simulink model "FM_Broadcast_Receiver"  (R2022a)
settings: Solver=FixedStepDiscrete  StartTime=0.0  StopTime=inf  RelTol=1e-3
PreLoadFcn:
  | addpath('matlab/broadcast');
undefined symbols (not defined in the file): fdesignblkfcn, gcbh
libraries: dspsigops x4, dsparch4 x4, dspsnks4 x1, sdrrlib x1
settings Model: Creator=Kate  LastModifiedBy=vovan
settings SolverCC: AlgebraicLoopSolver=TrustRegion
settings DebuggingCC: UnconnectedInputMsg=warning  UnconnectedOutputMsg=warning  UnconnectedLineMsg=warning  SFMachineParentedDataDiag=warning
settings SFSimCC: CustomCodeUndefinedFunction=UseInterfaceOnly

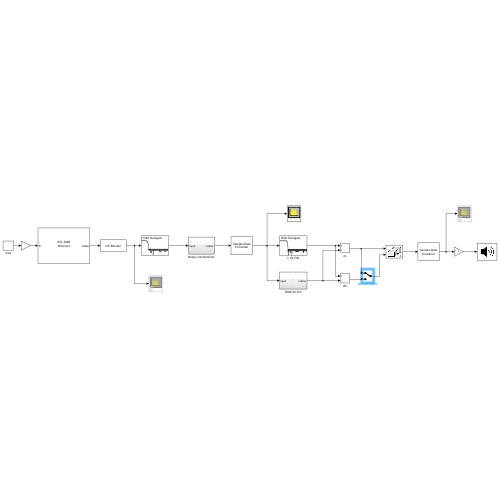
[thumbnail: Simulink's stored preview of the top-level diagram]
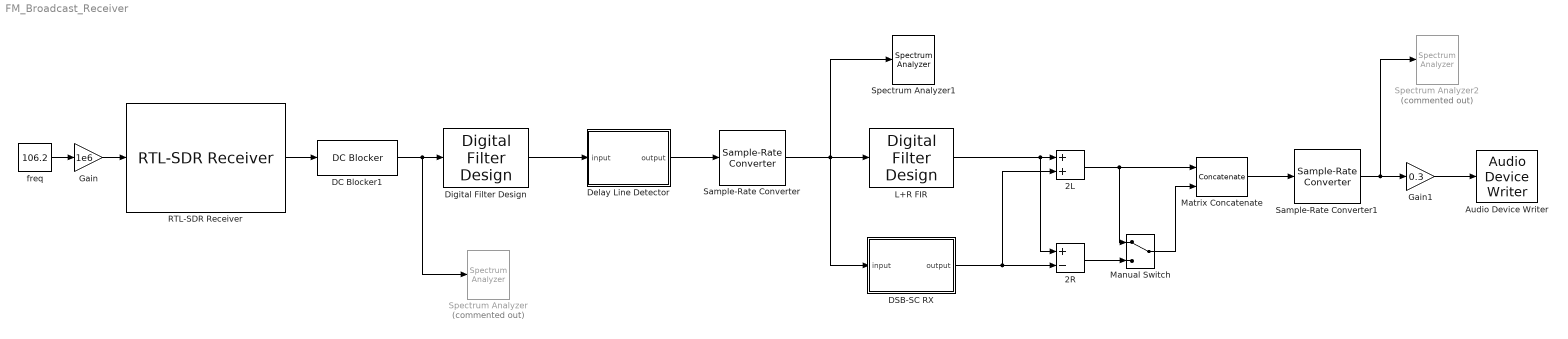
== system FM_Broadcast_Receiver ==
  2L : Sum
  2R : Sum  Inputs=+-
  Audio Device Writer : dspsnks4/Audio Device Writer  Driver=ALSA  Device=Default  InheritSampleRate=on  SampleRate=44100  BitDepth=16-bit integer  BufferSize=4096  NumBuffers=10  DefaultOutputChannelMapping=on  OutputChannelMapping=1:2  OutputNumUnderrunSamples=off  DriverIdx=8  DeviceWarnFlag=''
  DC Blocker1 : dspsigops/DC Blocker  Algorithm=IIR  NormalizedBandwidth=0.001  Length=50  Order=6  SimulateUsing=Code generation
      settings: SourceProductBaseCode=DS
  DSB-SC RX : Subsystem
  Delay Line Detector : Subsystem
  Digital Filter Design : dsparch4/Digital Filter Design  mwdsp_browser_bugfix_var=off
  Gain : Gain  Gain=1e6
  Gain1 : Gain  Gain=0.3
  L+R FIR : dsparch4/Digital Filter Design  mwdsp_browser_bugfix_var=off
  Manual Switch : ManualSwitch
  Matrix Concatenate : Concatenate  Mode=Multidimensional array  ConcatenateDimension=2
  RTL-SDR Receiver : sdrrlib/RTL-SDR Receiver  IPAddress=0  CenterFrequencySource=Input port  CenterFrequency=102.5e6  GainSource=AGC  Gain=0  ADCRate=1.2e6  FrequencyCorrection=0  LostSamplesOutputPort=off  LatencyOutputPort=off  OutputDataType=double  FrameLength=512*25  EnableBurstMode=off  NumFramesInBurst=20  sobjType=sdrr.internal.SDRRTLReceiverSL  dataUDPPort=-1  ctrlUDPPort=-1  subDeviceList=nosubdev  sdrBlockType=SDRBlockTypeSLT.SDRRxBlock  requester=UNUSED_BY_SFCN  sdrExecutionMode=SDRExecutionModeSLT.ExecModeHW  BypassUserLogic=off  DecimatorSelect=DDC decimator  SourceSelect=RF data  SineAmplitude=16000  EnableInternalClock=off  BypassIQBalance=off  IFBandwidth=40e6  ADCRateSource=Dialog  IntermediateFrequency=0  DecimationFactorSource=Dialog  DecimationFactor=512  RFFrequencyIsTunable=logical(1)  SampleTime=(512*25)/(1.2e6)  IFBandwidthSource=Dialog  SineFrequency=30000  BypassDCBlockingFilter=off  IntermediateFrequencySource=Dialog  IQBalanceCoefficients=64  SkipAllHardwareResetAndInitialization=off  EnableIQCalibrationTable=on  CacheIQCalibrationTable=off  EnableOffsetTuning=off  EnableRTLAGC=off  EnableTestMode=off  EnableTunerAGC=on  FrequencyCorrectionSource=Dialog  NumMLBuffers=128  NumUSBBuffers=16  RTLCrystalFrequency=28800000  TunerCrystalFrequency=28800000
      settings: SourceProductBaseCode=RTLSDR
  Sample-Rate Converter : dspsigops/Sample-Rate Converter  InputSampleRate=1.2e6  OutputSampleRate=1.2e5  OutputRateTolerance=0  Bandwidth=1.1e5  StopbandAttenuation=80  SimulateUsing=Code generation
      settings: SourceProductBaseCode=DS
  Sample-Rate Converter1 : dspsigops/Sample-Rate Converter  InputSampleRate=1.2e5  OutputSampleRate=48e3  OutputRateTolerance=0  Bandwidth=30e3  StopbandAttenuation=80  SimulateUsing=Code generation
      settings: SourceProductBaseCode=DS
  Spectrum Analyzer : SpectrumAnalyzer  Commented=on
  Spectrum Analyzer1 : SpectrumAnalyzer
  Spectrum Analyzer2 : SpectrumAnalyzer  Commented=on
  freq : Constant  Value=106.2
  wires:
  freq/1 -> Gain/1
  Gain/1 -> RTL-SDR Receiver/1
  Gain1/1 -> Audio Device Writer/1
  RTL-SDR Receiver/1 -> DC Blocker1/1
  DC Blocker1/1 -> Spectrum Analyzer/1, Digital Filter Design/1
  Sample-Rate Converter1/1 -> Spectrum Analyzer2/1, Gain1/1
  Digital Filter Design/1 -> Delay Line Detector/1(input)
  Delay Line Detector/1(output) -> Sample-Rate Converter/1
  Sample-Rate Converter/1 -> Spectrum Analyzer1/1, L+R FIR/1, DSB-SC RX/1(input)
  L+R FIR/1 -> 2R/1, 2L/1
  2L/1 -> Manual Switch/1, Matrix Concatenate/1
  Matrix Concatenate/1 -> Sample-Rate Converter1/1
  2R/1 -> Manual Switch/2
  Manual Switch/1 -> Matrix Concatenate/2
  DSB-SC RX/1(output) -> 2R/2, 2L/2

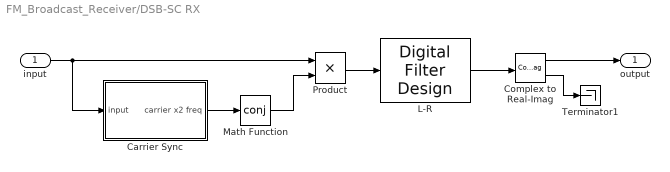
== system FM_Broadcast_Receiver/DSB-SC RX ==
  input : Inport
  Carrier Sync : Subsystem
  Complex to Real-Imag : ComplexToRealImag
  L-R : dsparch4/Digital Filter Design  mwdsp_browser_bugfix_var=off
  Math Function : Math  Operator=conj
  Product : Product
  Terminator1 : Terminator
  output : Outport
  wires:
  Carrier Sync/1(carrier x2 freq) -> Math Function/1
  Complex to Real-Imag/2 -> Terminator1/1
  L-R/1 -> Complex to Real-Imag/1
  Math Function/1 -> Product/2
  Complex to Real-Imag/1 -> output/1
  Product/1 -> L-R/1
  input/1 -> Product/1, Carrier Sync/1(input)

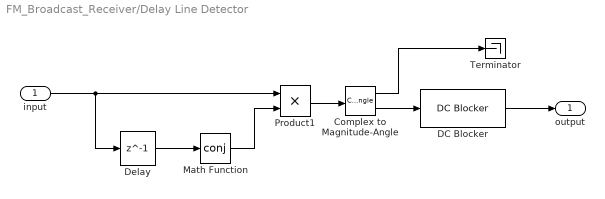
== system FM_Broadcast_Receiver/Delay Line Detector ==
  input : Inport
  Complex to Magnitude-Angle : ComplexToMagnitudeAngle
  DC Blocker : dspsigops/DC Blocker  Algorithm=IIR  NormalizedBandwidth=0.001  Length=50  Order=6  SimulateUsing=Code generation
      settings: SourceProductBaseCode=DS
  Delay : Delay  DelayLength=1  InputProcessing=Columns as channels (frame based)
  Math Function : Math  Operator=conj  SignedPower=on
  Product1 : Product
  Terminator : Terminator
  output : Outport
  wires:
  Complex to Magnitude-Angle/1 -> Terminator/1
  Math Function/1 -> Product1/2
  Complex to Magnitude-Angle/2 -> DC Blocker/1
  Delay/1 -> Math Function/1
  input/1 -> Product1/1, Delay/1
  Product1/1 -> Complex to Magnitude-Angle/1
  DC Blocker/1 -> output/1

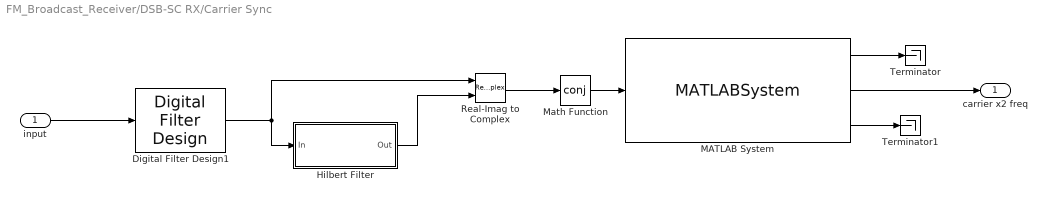
== system FM_Broadcast_Receiver/DSB-SC RX/Carrier Sync ==
  input : Inport
  Digital Filter Design1 : dsparch4/Digital Filter Design  mwdsp_browser_bugfix_var=off
  Hilbert Filter : Subsystem  DialogController=fdesignblkfcn  InitFcn=fdesignblkfcn(gcbh, {'InitFcn'});  mask(Hilbert Filter){}
      mask help: Design a Hilbert filter
      settings: CopyFcn=fdesignblkfcn(gcbh, {'CopyFcn'});
      mask Help: helpview(mapfilelocation('dsp'), 'dsphilbertfilter');
      mask Display: disp('Hilbert')
  MATLAB System : MATLABSystem  System=ComplexPLL  SampleFrequency=1.2e5  NoiseBandwidth=100  Dampingfactor=0.7  CentralFrequency=19e3  SimulateUsing=Code generation
      mask Type: ComplexPLL
      mask Display:
      | disp('ComplexPLL');
      | port_label('input',1,'InputFrame');
      | port_label('output',1,'OutputFrame');
      | port_label('output',2,'OutputFrameX2');
      | port_label('output',3,'FrequencyError');
  Math Function : Math  Operator=conj
  Real-Imag to Complex : RealImagToComplex
  Terminator : Terminator
  Terminator1 : Terminator
  carrier x2 freq : Outport
  wires:
  Math Function/1 -> MATLAB System/1
  Digital Filter Design1/1 -> Real-Imag to Complex/1, Hilbert Filter/1(In)
  Hilbert Filter/1(Out) -> Real-Imag to Complex/2
  MATLAB System/3 -> Terminator1/1
  MATLAB System/2 -> carrier x2 freq/1
  MATLAB System/1 -> Terminator/1
  Real-Imag to Complex/1 -> Math Function/1
  input/1 -> Digital Filter Design1/1

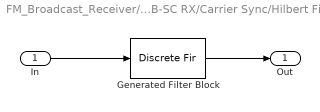
== system FM_Broadcast_Receiver/DSB-SC RX/Carrier Sync/Hilbert Filter ==
  In : Inport
  Generated Filter Block : DiscreteFir  Tag=BlockMethodSubSystem  Coefficients=[-0.00601736991412442357 -0.00193446246760335672 -0.00854710962923861325 -0.0046822849668463791 -0.0144315439127251088 -0.00938712195615788725 -0.0228599593847435417 -0.0171356232787936158 -0.0351510375097009997 -0.0301258171237506478 -0.054518552180406632 -0.0542241883804142621 -0.0918926908994361358 -0.113951243145950565 -0.217556697557992784 -0.627039254831127213 0.627039254831127213 0.217556697557992784 0.113951243145950565 0.0918926908994361358 0.0542241883804142621 0.054518552180406632 0.0301258171237506478 0.0351510375097009997 0.0171356232787936158 0.0228599593847435417 0.00938712195615788725 0.0144315439127251088 0.0046822849668463791 0.00854710962923861325 0.00193446246760335672 0.00601736991412442357]  InputProcessing=Columns as channels (frame based)
  Out : Outport  VectorParamsAs1DForOutWhenUnconnected=off
  wires:
  Generated Filter Block/1 -> Out/1
  In/1 -> Generated Filter Block/1
